simulink model "MBD_Function_Call_Subsystem"  (R2021b)
settings: Solver=FixedStepDiscrete  StartTime=0.0  StopTime=10.0  FixedStep=0.001  RelTol=1e-3
libraries: simulink x3
settings Model: Creator=waleed.elshemy  LastModifiedBy=waleed.elshemy
settings OptimizationCC: DefaultParameterBehavior=Inlined  UseDivisionForNetSlopeComputation=on  GainParamInheritBuiltInType=on  UseFloatMulNetSlope=on  InlineInvariantSignals=on  PassReuseOutputArgsAs=Individual arguments  ZeroExternalMemoryAtStartup=off  ZeroInternalMemoryAtStartup=off  NoFixptDivByZeroProtection=on  EfficientFloat2IntCast=on  LifeSpan=1  OptimizeBlockOrder=speed  DifferentSizesBufferReuse=on  EfficientTunableParamExpr=on
settings DebuggingCC: ParameterTunabilityLossMsg=error
settings HardwareCC: ProdLongLongMode=on
settings SFSimCC: MATLABDynamicMemAlloc=off
settings RTWCC: Description=Embedded Coder  SystemTargetFile=ert.tlc  TemplateMakefile=ert_default_tmf
settings CodeAppCC: ForceParamTrailComments=on  IgnoreCustomStorageClasses=off  OperatorAnnotations=on  SimulinkDataObjDesc=on  SFDataObjDesc=on  CustomSymbolStrGlobalVar=rt$N$M  CustomSymbolStrType=$N$M  CustomSymbolStrFcn=$N$M$F  CustomSymbolStrMacro=$N$M  InsertBlockDesc=on
settings ERTTargetCC: TargetLangStandard=C99 (ISO)  GenerateSampleERTMain=on  IncludeMdlTerminateFcn=off  CombineSignalStateStructs=on  SuppressErrorStatus=on  SupportAbsoluteTime=off  CodeInterfacePackaging=Reusable function  SupportComplex=off  InlinedParameterPlacement=NonHierarchical  ERTCustomFileTemplate=example_file_process.tlc

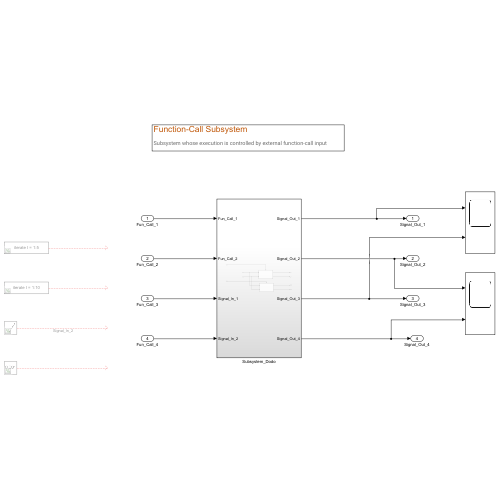
[thumbnail: Simulink's stored preview of the top-level diagram]
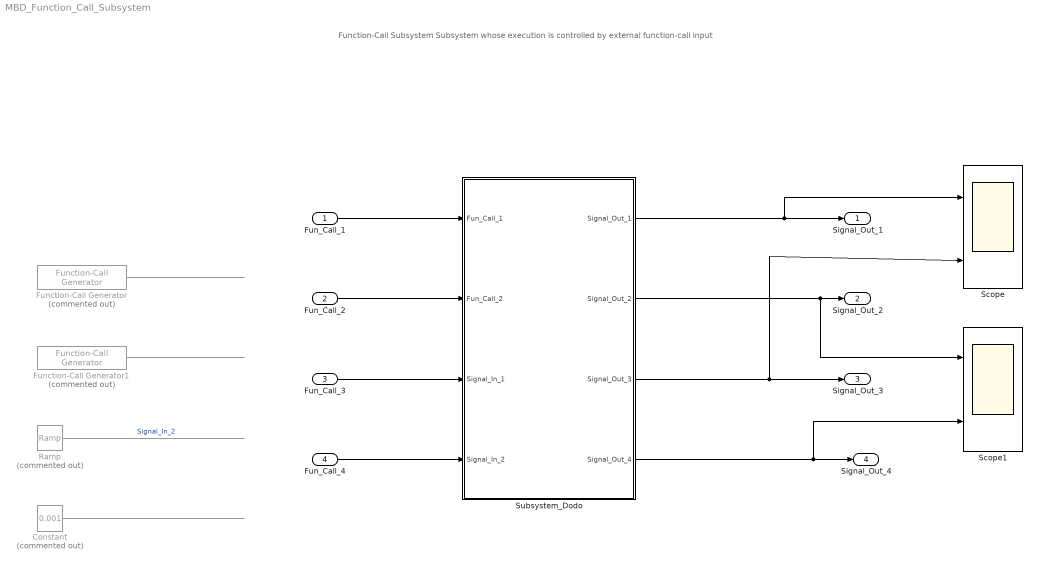
== system MBD_Function_Call_Subsystem ==
  note: Function-Call Subsystem
      | Subsystem whose execution is controlled by external function-call input
  Fun_Call_1 : Inport  OutputFunctionCall=on
  Fun_Call_2 : Inport  Port=2  OutputFunctionCall=on
  Fun_Call_3 : Inport  Port=3
  Fun_Call_4 : Inport  Port=4
  Constant : Constant  Commented=on  Value=0.001
  Function-Call Generator : simulink/Ports & Subsystems/Function-Call Generator  Commented=on  sample_time=1  numberOfIterations=5  DisallowWideOutput=off
  Function-Call Generator1 : simulink/Ports & Subsystems/Function-Call Generator  Commented=on  sample_time=1  numberOfIterations=10  DisallowWideOutput=off
  Ramp : simulink/Sources/Ramp  Commented=on  slope=0.01  start=0  InitialOutput=0
  Scope : Scope  NumInputPorts=2
  Scope1 : Scope  NumInputPorts=2
  Subsystem_Dodo : Subsystem
  Signal_Out_1 : Outport
  Signal_Out_2 : Outport  Port=2
  Signal_Out_3 : Outport  Port=3
  Signal_Out_4 : Outport  Port=4
  wires:
  Subsystem_Dodo/1(Signal_Out_1) -> Scope/1, Signal_Out_1/1
  Subsystem_Dodo/2(Signal_Out_2) -> Scope1/1, Signal_Out_2/1
  Subsystem_Dodo/3(Signal_Out_3) -> Scope/2, Signal_Out_3/1
  Subsystem_Dodo/4(Signal_Out_4) -> Scope1/2, Signal_Out_4/1
  Function-Call Generator1/1 -> ?
  Function-Call Generator/1 -> ?
  Ramp/1 -> ?  "Signal_In_2"
  Constant/1 -> ?
  Fun_Call_1/1 -> Subsystem_Dodo/1(Fun_Call_1)
  Fun_Call_2/1 -> Subsystem_Dodo/2(Fun_Call_2)
  Fun_Call_3/1 -> Subsystem_Dodo/3(Signal_In_1)
  Fun_Call_4/1 -> Subsystem_Dodo/4(Signal_In_2)

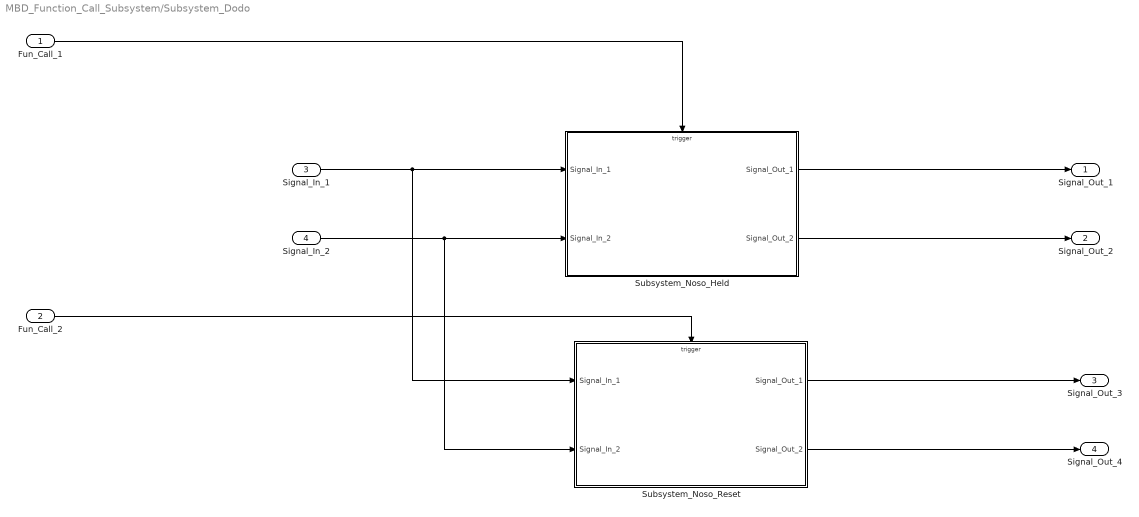
== system MBD_Function_Call_Subsystem/Subsystem_Dodo ==
  Fun_Call_1 : Inport
  Fun_Call_2 : Inport  Port=2
  Signal_In_1 : Inport  Port=3
  Signal_In_2 : Inport  Port=4
  Subsystem_Noso_Held : Subsystem  TreatAsAtomicUnit=on
  Subsystem_Noso_Reset : Subsystem  TreatAsAtomicUnit=on
      settings: RTWFileNameOpts=Use function name
  Signal_Out_1 : Outport
  Signal_Out_2 : Outport  Port=2
  Signal_Out_3 : Outport  Port=3
  Signal_Out_4 : Outport  Port=4
  wires:
  Subsystem_Noso_Held/1(Signal_Out_1) -> Signal_Out_1/1
  Signal_In_1/1 -> Subsystem_Noso_Reset/1(Signal_In_1), Subsystem_Noso_Held/1(Signal_In_1)
  Signal_In_2/1 -> Subsystem_Noso_Reset/2(Signal_In_2), Subsystem_Noso_Held/2(Signal_In_2)
  Subsystem_Noso_Held/2(Signal_Out_2) -> Signal_Out_2/1
  Subsystem_Noso_Reset/1(Signal_Out_1) -> Signal_Out_3/1
  Subsystem_Noso_Reset/2(Signal_Out_2) -> Signal_Out_4/1
  Fun_Call_1/1 -> Subsystem_Noso_Held/Trigger
  Fun_Call_2/1 -> Subsystem_Noso_Reset/Trigger

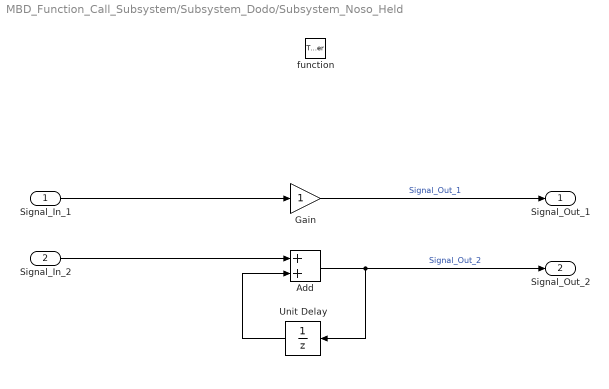
== system MBD_Function_Call_Subsystem/Subsystem_Dodo/Subsystem_Noso_Held ==
  Signal_In_1 : Inport
  Signal_In_2 : Inport  Port=2
  function : TriggerPort  TriggerType=function-call  VariantControl=(inherit)
  Add : Sum
  Gain : Gain
  Unit Delay : UnitDelay  SampleTime=-1  HasFrameUpgradeWarning=on
  Signal_Out_1 : Outport
  Signal_Out_2 : Outport  Port=2
  wires:
  Add/1 -> Signal_Out_2/1, Unit Delay/1  "Signal_Out_2"
  Gain/1 -> Signal_Out_1/1  "Signal_Out_1"
  Signal_In_2/1 -> Add/1
  Unit Delay/1 -> Add/2
  Signal_In_1/1 -> Gain/1

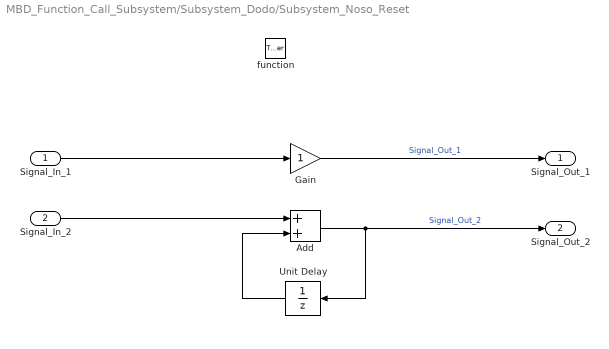
== system MBD_Function_Call_Subsystem/Subsystem_Dodo/Subsystem_Noso_Reset ==
  Signal_In_1 : Inport
  Signal_In_2 : Inport  Port=2
  function : TriggerPort  TriggerType=function-call  VariantControl=(inherit)  StatesWhenEnabling=reset
  Add : Sum
  Gain : Gain
  Unit Delay : UnitDelay  SampleTime=-1  HasFrameUpgradeWarning=on
  Signal_Out_1 : Outport
  Signal_Out_2 : Outport  Port=2
  wires:
  Signal_In_1/1 -> Gain/1
  Unit Delay/1 -> Add/2
  Signal_In_2/1 -> Add/1
  Gain/1 -> Signal_Out_1/1  "Signal_Out_1"
  Add/1 -> Unit Delay/1, Signal_Out_2/1  "Signal_Out_2"
